simulink model "adrc_han_new"  (R2021a)
settings: Solver=FixedStepDiscrete  StartTime=0.0  StopTime=100  FixedStep=0.001  RelTol=1e-3
undefined symbols (not defined in the file or in its folder): alpha1, alpha2, b, beta01, beta02, beta03, delta1, delta2, DiscIntNeverNeededParam, h, r0
settings Model: Creator=onqi  LastModifiedBy=onqi

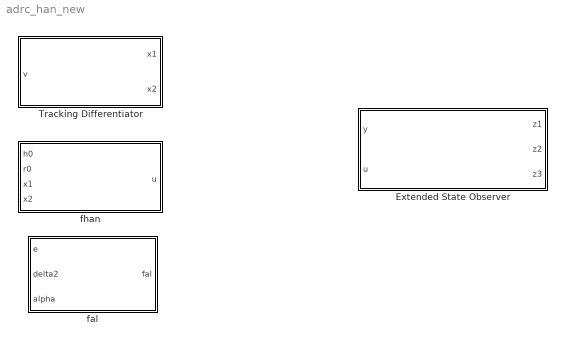
== system adrc_han_new ==
  Extended State Observer : Subsystem
      mask DialogControl fe1 Prompt: fal1(.) = fe1
      mask Display:
      | disp('Extended State Observer', 'texmode', 'on')
      | port_label('input', 1, 'y', 'texmode', 'on');
      | port_label('input', 2, 'u', 'texmode', 'on');
      | port_label('output', 1, 'z_1', 'texmode', 'on');
      | port_label('output', 2, 'z_2', 'texmode', 'on');
      | 
      | port_label('output', 3, 'z_3', 'texmode', 'on');
  Tracking Differentiator : Subsystem  SystemSampleTime=SystemSampleTime  mask{r0=50, h0=10, SystemSampleTime=-1}
      mask prompts: r0 "Tracking speed r0"; h0 "Tracking smoothness h0"; SystemSampleTime "Simulink:blkprm_prompts:AllBlksSampleTime"
      mask init:
      | h = str2num(get_param(gcs,'FixedStep'));
      mask TypeOptions SystemSampleTime: SystemSampleTime
      mask DialogControl SystemSampleTime Prompt: Sample time (-1 for inherited):
      mask Display:
      | disp('Tracking Differentiator')
      | port_label('input', 1, '\vee', 'texmode', 'on');
      | port_label('output', 1, 'x_1', 'texmode', 'on');
      | port_label('output', 2, '\Deltax_1', 'texmode', 'on');
  fal : Subsystem
      mask Display:
      | disp('fal(e, \alpha, \delta)', 'texmode', 'on')
      | port_label('input', 1, 'e', 'texmode', 'on');
      | port_label('output', 1, 'fal', 'texmode', 'on');
      | port_label('input', 2, '\delta', 'texmode', 'on');
      | port_label('input', 3, '\alpha', 'texmode', 'on');
  fhan : Subsystem
      mask Display:
      | disp('fhan(x_1, x_2, r, h)', 'texmode', 'on')
      | port_label('input', 1, 'h_0', 'texmode', 'on');
      | port_label('input', 2, 'r_0', 'texmode', 'on');
      | port_label('input', 3, 'x_1', 'texmode', 'on');
      | port_label('input', 4, 'x_2', 'texmode', 'on');
      | 
      | port_label('output', 1, 'f_{han}', 'texmode', 'on');

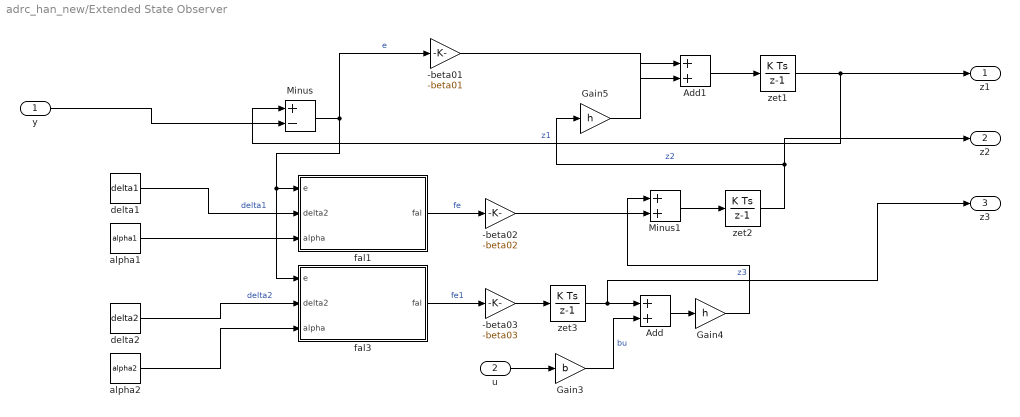
== system adrc_han_new/Extended State Observer ==
  y : Inport
  u : Inport  Port=2
  -beta01 : Gain  Gain=-beta01
  -beta02 : Gain  Gain=-beta02
  -beta03 : Gain  Gain=-beta03
  Add : Sum
  Add1 : Sum
  Gain3 : Gain  Gain=b
  Gain4 : Gain  Gain=h
  Gain5 : Gain  Gain=h
  Minus : Sum  Inputs=+-
  Minus1 : Sum
  alpha1 : Constant  Value=alpha1
  alpha2 : Constant  Value=alpha2
  delta1 : Constant  Value=delta1
  delta2 : Constant  Value=delta2
  fal1 : Subsystem
      mask Display:
      | disp('fal(e, \alpha, \delta)', 'texmode', 'on')
      | port_label('input', 1, 'e', 'texmode', 'on');
      | port_label('output', 1, 'fal', 'texmode', 'on');
      | port_label('input', 2, '\delta', 'texmode', 'on');
      | port_label('input', 3, '\alpha', 'texmode', 'on');
  fal3 : Subsystem
      mask Display:
      | disp('fal(e, \alpha, \delta)', 'texmode', 'on')
      | port_label('input', 1, 'e', 'texmode', 'on');
      | port_label('output', 1, 'fal', 'texmode', 'on');
      | port_label('input', 2, '\delta', 'texmode', 'on');
      | port_label('input', 3, '\alpha', 'texmode', 'on');
  zet1 : DiscreteIntegrator  SampleTime=-1  ICPrevOutput=DiscIntNeverNeededParam  ICPrevScaledInput=DiscIntNeverNeededParam
  zet2 : DiscreteIntegrator  SampleTime=-1  ICPrevOutput=DiscIntNeverNeededParam  ICPrevScaledInput=DiscIntNeverNeededParam
  zet3 : DiscreteIntegrator  SampleTime=-1  ICPrevOutput=DiscIntNeverNeededParam  ICPrevScaledInput=DiscIntNeverNeededParam
  z1 : Outport
  z2 : Outport  Port=2
  z3 : Outport  Port=3
  wires:
  delta1/1 -> fal1/2(delta2)  "delta1"
  -beta01/1 -> Add1/2
  Minus1/1 -> zet2/1
  zet3/1 -> z3/1, Add/1  "z3"
  delta2/1 -> fal3/2(delta2)  "delta2"
  zet2/1 -> z2/1, Gain5/1  "z2"
  zet1/1 -> z1/1, Minus/1  "z1"
  Gain5/1 -> Add1/1
  y/1 -> Minus/2
  u/1 -> Gain3/1
  Minus/1 -> fal3/1(e), fal1/1(e), -beta01/1  "e"
  -beta03/1 -> zet3/1
  Gain4/1 -> Minus1/1
  Add1/1 -> zet1/1
  -beta02/1 -> Minus1/2
  Gain3/1 -> Add/2  "bu"
  fal3/1(fal) -> -beta03/1  "fe1"
  fal1/1(fal) -> -beta02/1  "fe"
  Add/1 -> Gain4/1
  alpha1/1 -> fal1/3(alpha)
  alpha2/1 -> fal3/3(alpha)

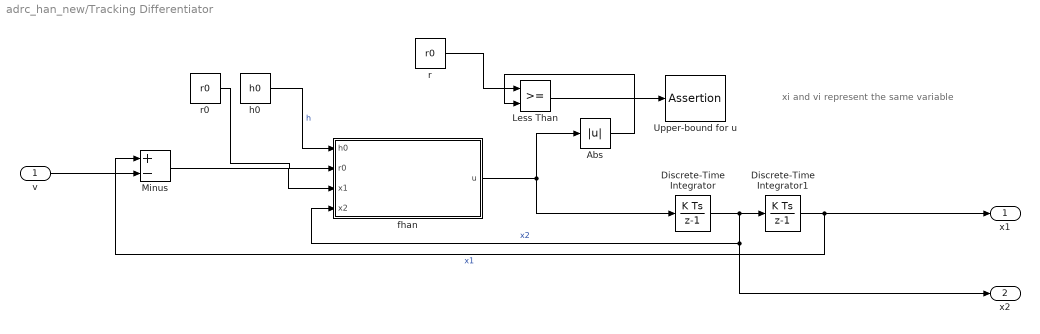
== system adrc_han_new/Tracking Differentiator ==
  note: xi and vi represent the same variable
  v : Inport
  Abs : Abs
  Discrete-Time Integrator : DiscreteIntegrator  SampleTime=-1  ICPrevOutput=DiscIntNeverNeededParam  ICPrevScaledInput=DiscIntNeverNeededParam
  Discrete-Time Integrator1 : DiscreteIntegrator  SampleTime=-1  ICPrevOutput=DiscIntNeverNeededParam  ICPrevScaledInput=DiscIntNeverNeededParam
  Less Than : RelationalOperator  OutDataTypeStr=boolean  RndMeth=Simplest
  Minus : Sum  Inputs=+-
  Upper-bound for u : Assertion
  fhan : Subsystem
  h0 : Constant  Value=h0  SampleTime=-1
  r : Constant  Value=r0  SampleTime=-1
  r0 : Constant  Value=r0  SampleTime=-1
  x1 : Outport
  x2 : Outport  Port=2
  wires:
  Abs/1 -> Less Than/2
  Less Than/1 -> Upper-bound for u/1
  Discrete-Time Integrator1/1 -> x1/1, Minus/1  "x1"
  Discrete-Time Integrator/1 -> fhan/4(x2), x2/1, Discrete-Time Integrator1/1  "x2"
  v/1 -> Minus/2
  r/1 -> Less Than/1
  fhan/1(u) -> Discrete-Time Integrator/1, Abs/1
  h0/1 -> fhan/1(h0)  "h"
  r0/1 -> fhan/2(r0)
  Minus/1 -> fhan/3(x1)

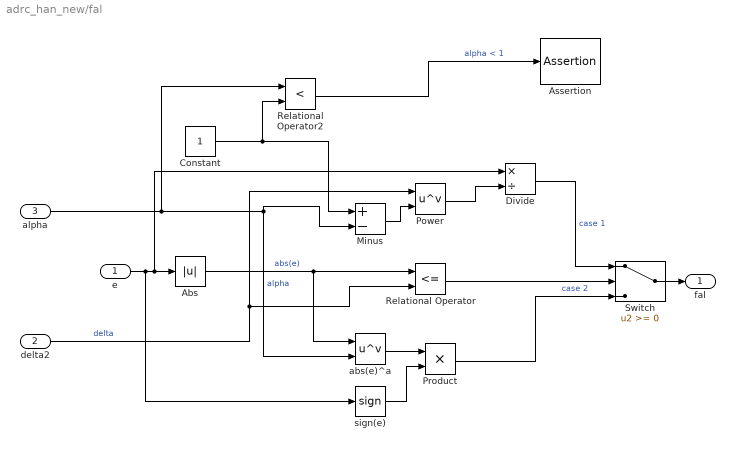
== system adrc_han_new/fal ==
  e : Inport
  delta2 : Inport  Port=2
  alpha : Inport  Port=3
  Abs : Abs
  Assertion : Assertion
  Constant : Constant
  Divide : Product  Inputs=*/
  Minus : Sum  Inputs=+-
  Power : Math  Operator=pow  SaturateOnIntegerOverflow=on
  Product : Product
  Relational Operator : RelationalOperator  Operator=<=  OutDataTypeStr=boolean  RndMeth=Simplest
  Relational Operator2 : RelationalOperator  Operator=<  OutDataTypeStr=boolean  RndMeth=Simplest
  Switch : Switch
  abs(e)^a : Math  Operator=pow  SaturateOnIntegerOverflow=on
  sign(e) : Signum
  fal : Outport
  wires:
  sign(e)/1 -> Product/2
  Switch/1 -> fal/1
  Relational Operator/1 -> Switch/2
  Abs/1 -> abs(e)^a/1, Relational Operator/1  "abs(e)"
  Power/1 -> Divide/2
  alpha/1 -> Relational Operator2/1, Minus/2, abs(e)^a/2  "alpha"
  Minus/1 -> Power/2
  e/1 -> sign(e)/1, Divide/1, Abs/1
  abs(e)^a/1 -> Product/1
  Product/1 -> Switch/3  "case 2"
  Divide/1 -> Switch/1  "case 1"
  delta2/1 -> Relational Operator/2, Power/1  "delta"
  Constant/1 -> Relational Operator2/2, Minus/1
  Relational Operator2/1 -> Assertion/1  "alpha < 1"

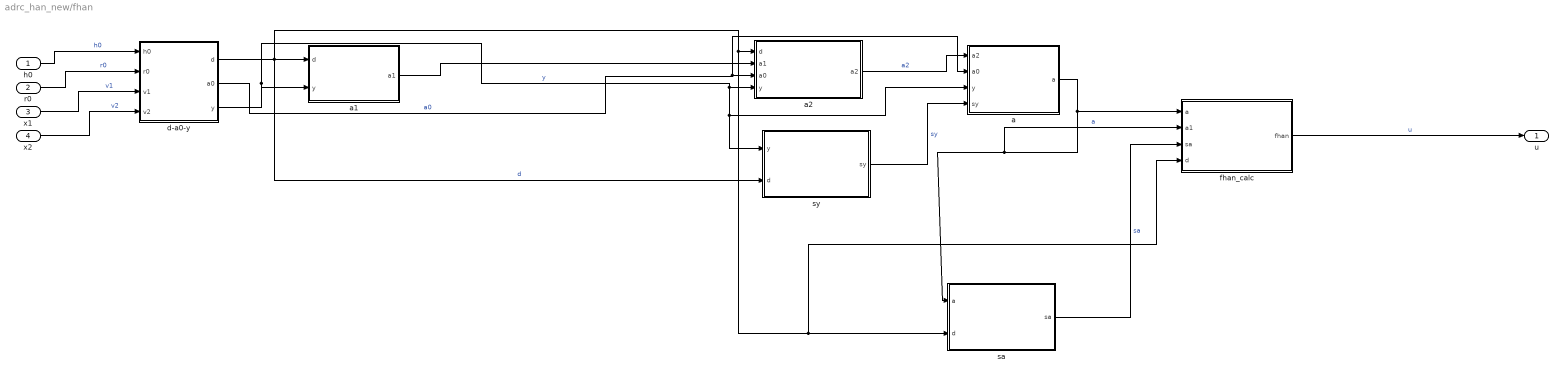
== system adrc_han_new/fhan ==
  h0 : Inport
  r0 : Inport  Port=2
  x1 : Inport  Port=3
  x2 : Inport  Port=4
  a : Subsystem
  a1 : Subsystem
  a2 : Subsystem
  d-a0-y : Subsystem
  fhan_calc : Subsystem
  sa : Subsystem
  sy : Subsystem
  u : Outport
  wires:
  h0/1 -> d-a0-y/1(h0)  "h0"
  r0/1 -> d-a0-y/2(r0)  "r0"
  x1/1 -> d-a0-y/3(v1)  "v1"
  x2/1 -> d-a0-y/4(v2)  "v2"
  d-a0-y/1(d) -> sy/2(d), a1/1(d), fhan_calc/4(d), sa/2(d), a2/1(d)  "d"
  d-a0-y/3(y) -> a/3(y), sy/1(y), a2/4(y), a1/2(y)  "y"
  a1/1(a1) -> a2/2(a1)
  d-a0-y/2(a0) -> a/2(a0), a2/3(a0)  "a0"
  a2/1(a2) -> a/1(a2)  "a2"
  sy/1(sy) -> a/4(sy)  "sy"
  a/1(a) -> sa/1(a), fhan_calc/2(a1), fhan_calc/1(a)  "a"
  sa/1(sa) -> fhan_calc/3(sa)  "sa"
  fhan_calc/1(fhan) -> u/1  "u"

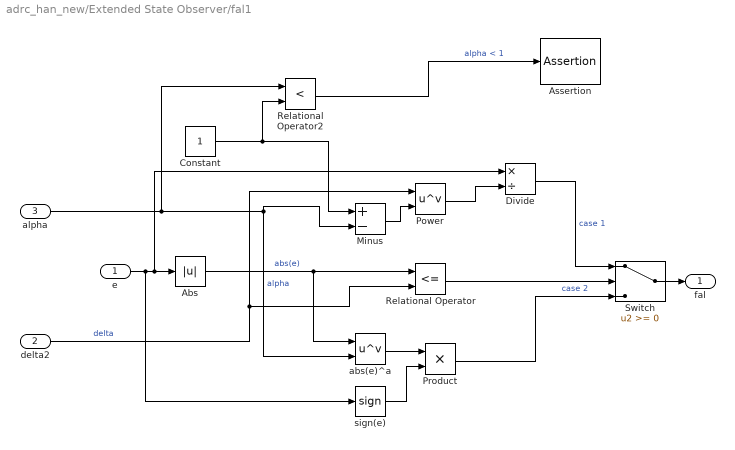
== system adrc_han_new/Extended State Observer/fal1 ==
  e : Inport
  delta2 : Inport  Port=2
  alpha : Inport  Port=3
  Abs : Abs
  Assertion : Assertion
  Constant : Constant
  Divide : Product  Inputs=*/
  Minus : Sum  Inputs=+-
  Power : Math  Operator=pow  SaturateOnIntegerOverflow=on
  Product : Product
  Relational Operator : RelationalOperator  Operator=<=  OutDataTypeStr=boolean  RndMeth=Simplest
  Relational Operator2 : RelationalOperator  Operator=<  OutDataTypeStr=boolean  RndMeth=Simplest
  Switch : Switch
  abs(e)^a : Math  Operator=pow  SaturateOnIntegerOverflow=on
  sign(e) : Signum
  fal : Outport
  wires:
  sign(e)/1 -> Product/2
  Switch/1 -> fal/1
  Relational Operator/1 -> Switch/2
  Abs/1 -> abs(e)^a/1, Relational Operator/1  "abs(e)"
  Power/1 -> Divide/2
  alpha/1 -> Relational Operator2/1, Minus/2, abs(e)^a/2  "alpha"
  Minus/1 -> Power/2
  e/1 -> sign(e)/1, Divide/1, Abs/1
  abs(e)^a/1 -> Product/1
  Product/1 -> Switch/3  "case 2"
  Divide/1 -> Switch/1  "case 1"
  delta2/1 -> Relational Operator/2, Power/1  "delta"
  Constant/1 -> Relational Operator2/2, Minus/1
  Relational Operator2/1 -> Assertion/1  "alpha < 1"

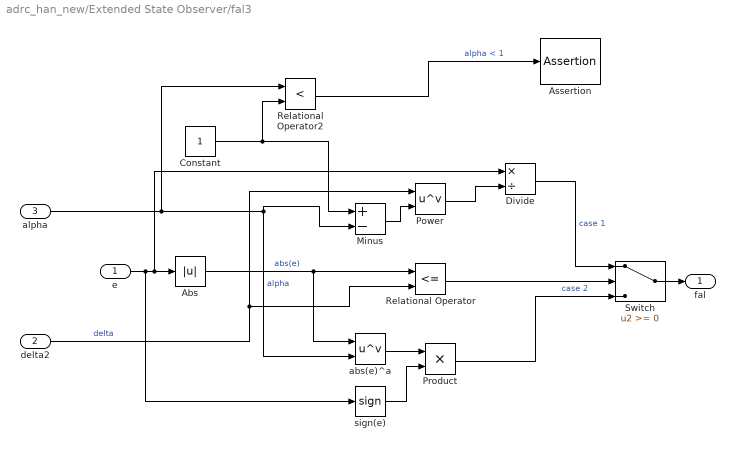
== system adrc_han_new/Extended State Observer/fal3 ==
  e : Inport
  delta2 : Inport  Port=2
  alpha : Inport  Port=3
  Abs : Abs
  Assertion : Assertion
  Constant : Constant
  Divide : Product  Inputs=*/
  Minus : Sum  Inputs=+-
  Power : Math  Operator=pow  SaturateOnIntegerOverflow=on
  Product : Product
  Relational Operator : RelationalOperator  Operator=<=  OutDataTypeStr=boolean  RndMeth=Simplest
  Relational Operator2 : RelationalOperator  Operator=<  OutDataTypeStr=boolean  RndMeth=Simplest
  Switch : Switch
  abs(e)^a : Math  Operator=pow  SaturateOnIntegerOverflow=on
  sign(e) : Signum
  fal : Outport
  wires:
  sign(e)/1 -> Product/2
  Switch/1 -> fal/1
  Relational Operator/1 -> Switch/2
  Abs/1 -> abs(e)^a/1, Relational Operator/1  "abs(e)"
  Power/1 -> Divide/2
  alpha/1 -> Relational Operator2/1, Minus/2, abs(e)^a/2  "alpha"
  Minus/1 -> Power/2
  e/1 -> sign(e)/1, Divide/1, Abs/1
  abs(e)^a/1 -> Product/1
  Product/1 -> Switch/3  "case 2"
  Divide/1 -> Switch/1  "case 1"
  delta2/1 -> Relational Operator/2, Power/1  "delta"
  Constant/1 -> Relational Operator2/2, Minus/1
  Relational Operator2/1 -> Assertion/1  "alpha < 1"

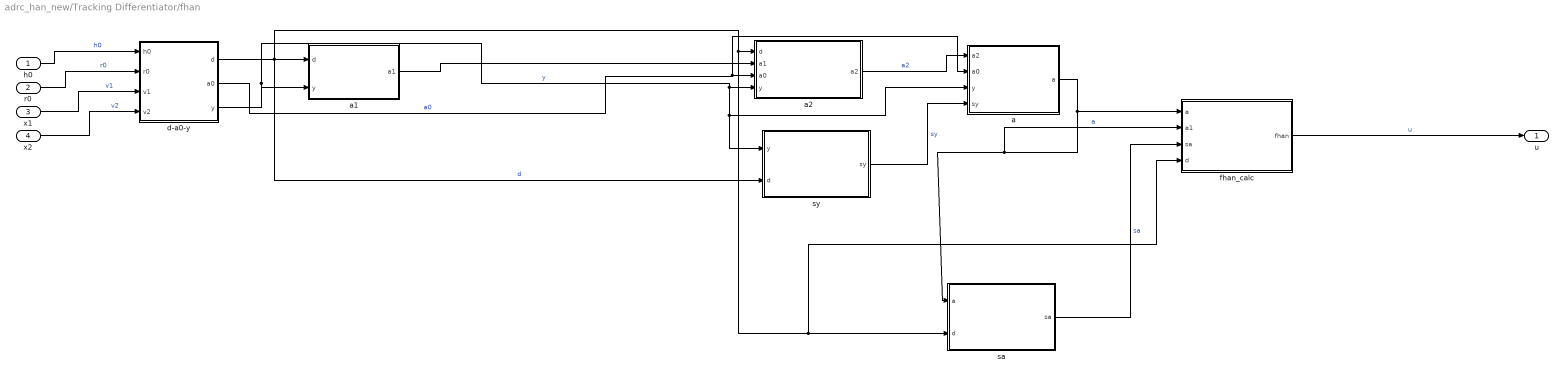
== system adrc_han_new/Tracking Differentiator/fhan ==
  h0 : Inport
  r0 : Inport  Port=2
  x1 : Inport  Port=3
  x2 : Inport  Port=4
  a : Subsystem
  a1 : Subsystem
  a2 : Subsystem
  d-a0-y : Subsystem
  fhan_calc : Subsystem
  sa : Subsystem
  sy : Subsystem
  u : Outport
  wires:
  h0/1 -> d-a0-y/1(h0)  "h0"
  r0/1 -> d-a0-y/2(r0)  "r0"
  x1/1 -> d-a0-y/3(v1)  "v1"
  x2/1 -> d-a0-y/4(v2)  "v2"
  d-a0-y/1(d) -> sy/2(d), a1/1(d), fhan_calc/4(d), sa/2(d), a2/1(d)  "d"
  d-a0-y/3(y) -> a/3(y), sy/1(y), a2/4(y), a1/2(y)  "y"
  a1/1(a1) -> a2/2(a1)
  d-a0-y/2(a0) -> a/2(a0), a2/3(a0)  "a0"
  a2/1(a2) -> a/1(a2)  "a2"
  sy/1(sy) -> a/4(sy)  "sy"
  a/1(a) -> sa/1(a), fhan_calc/2(a1), fhan_calc/1(a)  "a"
  sa/1(sa) -> fhan_calc/3(sa)  "sa"
  fhan_calc/1(fhan) -> u/1  "u"

== system adrc_han_new/fhan/a ==
  a2 : Inport
  a0 : Inport  Port=2
  y : Inport  Port=3
  sy : Inport  Port=4
  Add : Sum  Inputs=++-
  Plus : Sum
  Product : Product
  a : Outport
  wires:
  y/1 -> Add/2
  a0/1 -> Add/1
  Plus/1 -> a/1  "a"
  a2/1 -> Plus/2, Add/3
  Product/1 -> Plus/1
  sy/1 -> Product/2
  Add/1 -> Product/1

== system adrc_han_new/fhan/a1 ==
  d : Inport
  y : Inport  Port=2
  Abs : Abs
  Add : Sum
  Gain : Gain  Gain=8
  Product : Product
  Sqrt : Sqrt  SaturateOnIntegerOverflow=on
  a1 : Outport
  wires:
  Product/1 -> Sqrt/1
  Sqrt/1 -> a1/1  "a1"
  y/1 -> Abs/1
  d/1 -> Product/1, Add/1
  Add/1 -> Product/2
  Abs/1 -> Gain/1
  Gain/1 -> Add/2  "8|y|"

== system adrc_han_new/fhan/a2 ==
  d : Inport
  a1 : Inport  Port=2
  a0 : Inport  Port=3
  y : Inport  Port=4
  Add : Sum
  Gain : Gain  Gain=1/2
  Minus : Sum  Inputs=+-
  Product : Product
  sign(y) : Signum
  a2 : Outport
  wires:
  sign(y)/1 -> Product/1  "sign(y)"
  Minus/1 -> Product/2  "a1 - d"
  Product/1 -> Gain/1
  y/1 -> sign(y)/1
  a0/1 -> Add/1
  d/1 -> Minus/2
  Add/1 -> a2/1  "a2"
  a1/1 -> Minus/1
  Gain/1 -> Add/2

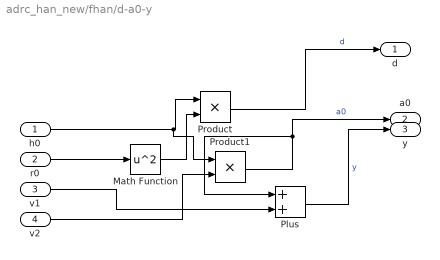
== system adrc_han_new/fhan/d-a0-y ==
  h0 : Inport
  r0 : Inport  Port=2
  v1 : Inport  Port=3
  v2 : Inport  Port=4
  Math Function : Math  Operator=square  SaturateOnIntegerOverflow=on
  Plus : Sum
  Product : Product
  Product1 : Product
  d : Outport
  a0 : Outport  Port=2
  y : Outport  Port=3
  wires:
  Math Function/1 -> Product/2
  v1/1 -> Plus/2
  Plus/1 -> y/1  "y"
  r0/1 -> Math Function/1
  Product1/1 -> a0/1, Plus/1  "a0"
  v2/1 -> Product1/2
  Product/1 -> d/1  "d"
  h0/1 -> Product1/1, Product/1

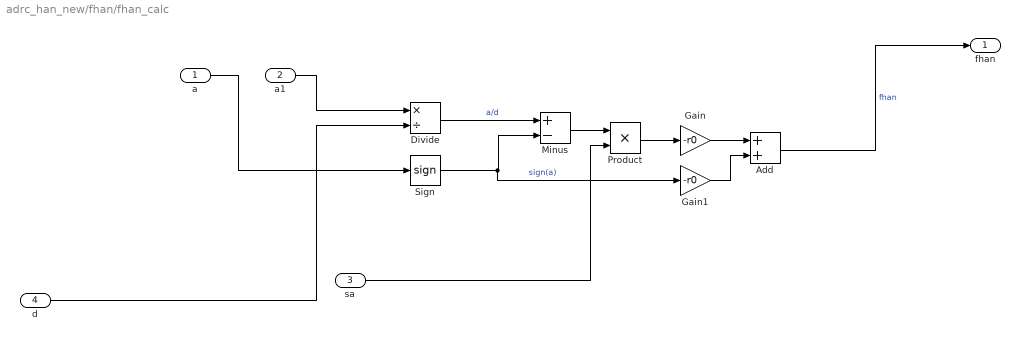
== system adrc_han_new/fhan/fhan_calc ==
  a : Inport
  a1 : Inport  Port=2
  sa : Inport  Port=3
  d : Inport  Port=4
  Add : Sum
  Divide : Product  Inputs=*/
  Gain : Gain  Gain=-r0
  Gain1 : Gain  Gain=-r0
  Minus : Sum  Inputs=+-
  Product : Product
  Sign : Signum
  fhan : Outport
  wires:
  sa/1 -> Product/2
  Minus/1 -> Product/1
  Gain/1 -> Add/1
  Divide/1 -> Minus/1  "a/d"
  a/1 -> Sign/1
  Add/1 -> fhan/1  "fhan"
  a1/1 -> Divide/1
  Gain1/1 -> Add/2
  d/1 -> Divide/2
  Product/1 -> Gain/1
  Sign/1 -> Gain1/1, Minus/2  "sign(a)"

== system adrc_han_new/fhan/sa ==
  a : Inport
  d : Inport  Port=2
  Gain : Gain  Gain=1/2
  Minus : Sum  Inputs=+-
  Minus1 : Sum  Inputs=+-
  Plus : Sum
  Sign1 : Signum
  Sign2 : Signum
  sa : Outport
  wires:
  Sign1/1 -> Minus1/1
  Plus/1 -> Sign1/1
  a/1 -> Minus/1, Plus/1
  Sign2/1 -> Minus1/2
  Minus/1 -> Sign2/1
  Minus1/1 -> Gain/1
  d/1 -> Minus/2, Plus/2
  Gain/1 -> sa/1  "s"

== system adrc_han_new/fhan/sy ==
  y : Inport
  d : Inport  Port=2
  Gain : Gain  Gain=1/2
  Minus : Sum  Inputs=+-
  Minus1 : Sum  Inputs=+-
  Plus : Sum
  Sign1 : Signum
  Sign2 : Signum
  sy : Outport
  wires:
  Sign1/1 -> Minus1/1
  Plus/1 -> Sign1/1
  y/1 -> Minus/1, Plus/1
  Sign2/1 -> Minus1/2
  Minus/1 -> Sign2/1
  Minus1/1 -> Gain/1
  d/1 -> Minus/2, Plus/2
  Gain/1 -> sy/1  "s"

== system adrc_han_new/Tracking Differentiator/fhan/a ==
  a2 : Inport
  a0 : Inport  Port=2
  y : Inport  Port=3
  sy : Inport  Port=4
  Add : Sum  Inputs=++-
  Plus : Sum
  Product : Product
  a : Outport
  wires:
  y/1 -> Add/2
  a0/1 -> Add/1
  Plus/1 -> a/1  "a"
  a2/1 -> Plus/2, Add/3
  Product/1 -> Plus/1
  sy/1 -> Product/2
  Add/1 -> Product/1

== system adrc_han_new/Tracking Differentiator/fhan/a1 ==
  d : Inport
  y : Inport  Port=2
  Abs : Abs
  Add : Sum
  Gain : Gain  Gain=8
  Product : Product
  Sqrt : Sqrt  SaturateOnIntegerOverflow=on
  a1 : Outport
  wires:
  Product/1 -> Sqrt/1
  Sqrt/1 -> a1/1  "a1"
  y/1 -> Abs/1
  d/1 -> Product/1, Add/1
  Add/1 -> Product/2
  Abs/1 -> Gain/1
  Gain/1 -> Add/2  "8|y|"

== system adrc_han_new/Tracking Differentiator/fhan/a2 ==
  d : Inport
  a1 : Inport  Port=2
  a0 : Inport  Port=3
  y : Inport  Port=4
  Add : Sum
  Gain : Gain  Gain=1/2
  Minus : Sum  Inputs=+-
  Product : Product
  sign(y) : Signum
  a2 : Outport
  wires:
  sign(y)/1 -> Product/1  "sign(y)"
  Minus/1 -> Product/2  "a1 - d"
  Product/1 -> Gain/1
  y/1 -> sign(y)/1
  a0/1 -> Add/1
  d/1 -> Minus/2
  Add/1 -> a2/1  "a2"
  a1/1 -> Minus/1
  Gain/1 -> Add/2

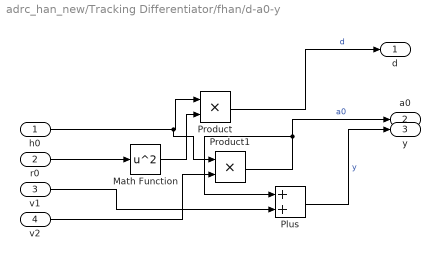
== system adrc_han_new/Tracking Differentiator/fhan/d-a0-y ==
  h0 : Inport
  r0 : Inport  Port=2
  v1 : Inport  Port=3
  v2 : Inport  Port=4
  Math Function : Math  Operator=square  SaturateOnIntegerOverflow=on
  Plus : Sum
  Product : Product
  Product1 : Product
  d : Outport
  a0 : Outport  Port=2
  y : Outport  Port=3
  wires:
  Math Function/1 -> Product/2
  v1/1 -> Plus/2
  Plus/1 -> y/1  "y"
  r0/1 -> Math Function/1
  Product1/1 -> a0/1, Plus/1  "a0"
  v2/1 -> Product1/2
  Product/1 -> d/1  "d"
  h0/1 -> Product1/1, Product/1

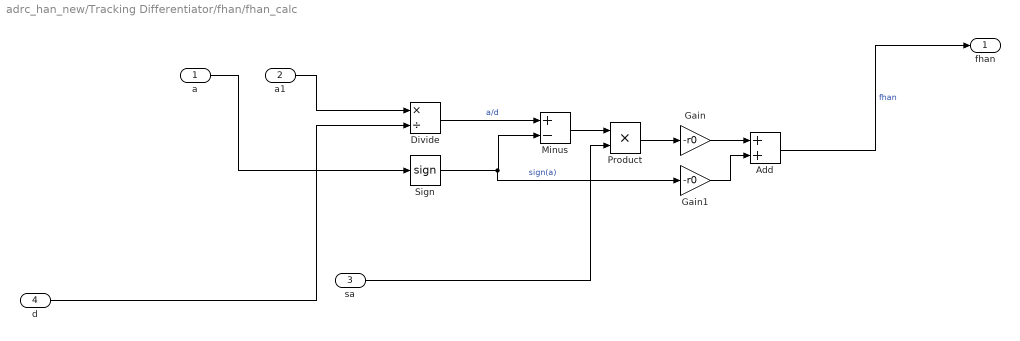
== system adrc_han_new/Tracking Differentiator/fhan/fhan_calc ==
  a : Inport
  a1 : Inport  Port=2
  sa : Inport  Port=3
  d : Inport  Port=4
  Add : Sum
  Divide : Product  Inputs=*/
  Gain : Gain  Gain=-r0
  Gain1 : Gain  Gain=-r0
  Minus : Sum  Inputs=+-
  Product : Product
  Sign : Signum
  fhan : Outport
  wires:
  sa/1 -> Product/2
  Minus/1 -> Product/1
  Gain/1 -> Add/1
  Divide/1 -> Minus/1  "a/d"
  a/1 -> Sign/1
  Add/1 -> fhan/1  "fhan"
  a1/1 -> Divide/1
  Gain1/1 -> Add/2
  d/1 -> Divide/2
  Product/1 -> Gain/1
  Sign/1 -> Gain1/1, Minus/2  "sign(a)"

== system adrc_han_new/Tracking Differentiator/fhan/sa ==
  a : Inport
  d : Inport  Port=2
  Gain : Gain  Gain=1/2
  Minus : Sum  Inputs=+-
  Minus1 : Sum  Inputs=+-
  Plus : Sum
  Sign1 : Signum
  Sign2 : Signum
  sa : Outport
  wires:
  Sign1/1 -> Minus1/1
  Plus/1 -> Sign1/1
  a/1 -> Minus/1, Plus/1
  Sign2/1 -> Minus1/2
  Minus/1 -> Sign2/1
  Minus1/1 -> Gain/1
  d/1 -> Minus/2, Plus/2
  Gain/1 -> sa/1  "s"

== system adrc_han_new/Tracking Differentiator/fhan/sy ==
  y : Inport
  d : Inport  Port=2
  Gain : Gain  Gain=1/2
  Minus : Sum  Inputs=+-
  Minus1 : Sum  Inputs=+-
  Plus : Sum
  Sign1 : Signum
  Sign2 : Signum
  sy : Outport
  wires:
  Sign1/1 -> Minus1/1
  Plus/1 -> Sign1/1
  y/1 -> Minus/1, Plus/1
  Sign2/1 -> Minus1/2
  Minus/1 -> Sign2/1
  Minus1/1 -> Gain/1
  d/1 -> Minus/2, Plus/2
  Gain/1 -> sy/1  "s"
